simulink model "Mil_Mirror_Subsystem"  (R2018a)
settings: Solver=VariableStepAuto  StartTime=0.0  StopTime=10.0  RelTol=1e-3
undefined symbols (not defined in the file or in its folder): sigbuilder_block
settings Model: Creator=99003191  LastModifiedBy=Anoosha Clarance
settings DataIOCC: ReturnWorkspaceOutputs=on
settings SFSimCC: SimUseLocalCustomCode=on
settings RTWCC: RTWUseLocalCustomCode=on

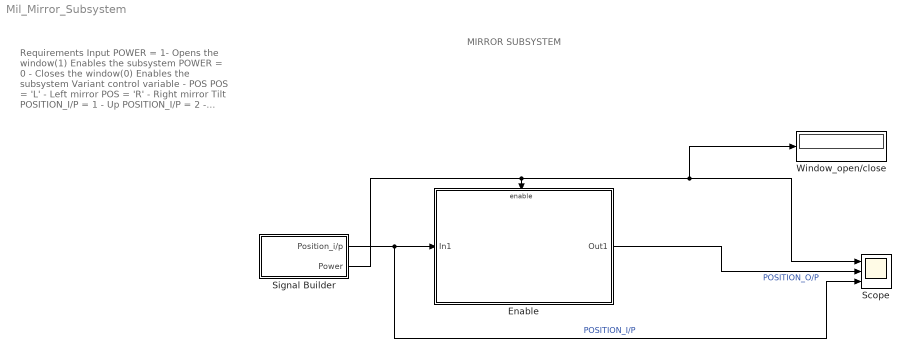
== system Mil_Mirror_Subsystem ==
  note: Requirements
      | Input
      | POWER = 1- Opens the window(1) Enables the subsystem
      | POWER = 0 - Closes the window(0) Enables the subsystem
      | Variant control variable - POS
      | POS = 'L' - Left mirror
      | POS = 'R' - Right mirror
      | Tilt
      | POSITION_I/P = 1 - Up
      | POSITION_I/P = 2 - Down
      | Pan
      | POSITION_I/P = 1 - Right
      | POSITION_I/P = 1 - Left
      |
      | Output
      | Tilt
      | POSITION_O/P = 11 - Left mirror Up
      | POSITION_O/P = 12 - Left mirror Down
      | POSITION_O/P = 21 - Right mirror Up
      | POSITION_O/P = 22 - Right mirror Down
      | Pan
      | POSITION_O/P = 13 - Left mirror Right
      | POSITION_O/P = 14 - Left mirror Left
      | POSITION_O/P = 23 - Right mirror Right
      | POSITION_O/P = 24 - Right mirror Left
  note: MIRROR SUBSYSTEM
  Enable : Subsystem  TreatAsAtomicUnit=on
  Scope : Scope  NumInputPorts=3
  Signal Builder : Subsystem  Tag=STV Subsys  LoadFcn=sigbuilder_block('load');  StartFcn=sigbuilder_block('start');  StopFcn=sigbuilder_block('stop');  ClipboardFcn=sigbuilder_block('clipboard');  mask(Sigbuilder block){tuvar=[0:10]}
      mask help: Simulink:masks:SigbuilderBlock_MD
      mask init:
      | if ~strcmp(get_param(bdroot(gcbh),'SimulationStatus'),'stopped') tuvar = sigbuilder_block('maskInit'); end
      settings: CopyFcn=sigbuilder_block('copy');  DeleteFcn=sigbuilder_block('delete');  ModelCloseFcn=sigbuilder_block('modelClose');  PreSaveFcn=sigbuilder_block('preSave');  PauseFcn=sigbuilder_block('pause');  ContinueFcn=sigbuilder_block('continue');  NameChangeFcn=sigbuilder_block('namechange');  OpenFcn=sigbuilder_block('open',[440.25 156.75 544.5 355.5 ]);  CloseFcn=sigbuilder_block('close');
      mask Display: plot(0, 0, 100, 100,[2, 2, 32, 32, 2], [68, 8, 8, 68, 68],[32, 2], [38, 38], [32, 19, 2],[53, 60, 44], [32, 17, 17, 2],[16, 16, 31, 31]);txt = getActiveGroup(gcbh);text(2, 100, txt,'verticalAlignment', 'top');
  Window_open/close : Display
  wires:
  Signal Builder/1(Position_i/p) -> Scope/3, Enable/1(In1)  "POSITION_I/P"
  Signal Builder/2(Power) -> Window_open/close/1, Scope/1, Enable/Enable
  Enable/1(Out1) -> Scope/2  "POSITION_O/P"

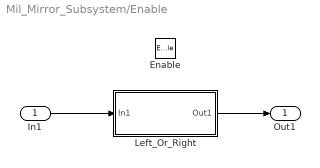
== system Mil_Mirror_Subsystem/Enable ==
  In1 : Inport
  Enable : EnablePort
  Left_Or_Right : Subsystem  Variant=on
  Out1 : Outport
  wires:
  In1/1 -> Left_Or_Right/1(In1)
  Left_Or_Right/1(Out1) -> Out1/1

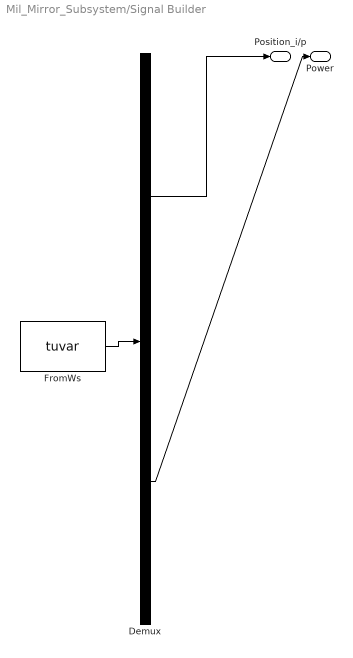
== system Mil_Mirror_Subsystem/Signal Builder ==
  Demux : Demux  Tag=STV Demux  Outputs=2
      settings: DisplayOption=none
  FromWs : FromWorkspace  Tag=STV FromWs  VariableName=tuvar
      SigBuilderData=|
      | common.afterFinalStr = 'Extrapolate'
      | common.sampleTime = 0
      | dataSet.timeRange = [0 10]
      | dataSet.name = 'Group 1'
      | sbobj.Groups.Name = 'Group 1'
      | sbobj.Groups.Signals(1).Name = 'Position_i/p'
      | sbobj.Groups.Signals(1).XData = [0 1 1 2 2 3.02 3.02 4.02 4.02 5 5 5.98 5.98 10]
      | sbobj.Groups.Signals(1).YData = [0 0 3 3 2 2 1 1 3 3 4 4 0 0]
      | sbobj.Groups.Signals(2).Name = 'Power'
      | sbobj.Groups.Signals(2).XData = [0 0.54 0.54 6 6 10]
      | sbobj.Groups.Signals(2).YData = [0 0 1 1 0 0]
  Position_i/p : Outport  Tag=STV Outport
  Power : Outport  Tag=STV Outport  Port=2
  wires:
  Demux/1 -> Position_i/p/1
  FromWs/1 -> Demux/1
  Demux/2 -> Power/1

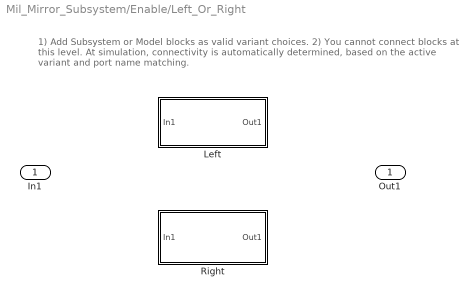
== system Mil_Mirror_Subsystem/Enable/Left_Or_Right ==
  note: 1) Add Subsystem or Model blocks as valid variant choices.
      | 2) You cannot connect blocks at this level. At simulation, connectivity is automatically
      | determined, based on the active variant and port name matching.
  In1 : Inport
  Left : Subsystem  VariantControl=POS == 'L'
  Right : Subsystem  VariantControl=POS == 'R'
  Out1 : Outport

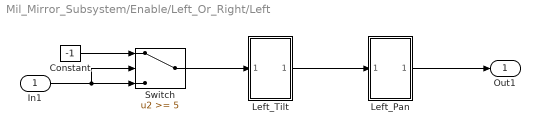
== system Mil_Mirror_Subsystem/Enable/Left_Or_Right/Left ==
  In1 : Inport
  Constant : Constant  Value=-1
  Left_Pan : Subsystem
  Left_Tilt : Subsystem
  Switch : Switch  Threshold=5
  Out1 : Outport
  wires:
  In1/1 -> Switch/2, Switch/3
  Constant/1 -> Switch/1
  Switch/1 -> Left_Tilt/1(In1)
  Left_Tilt/1(Out1) -> Left_Pan/1(In1)
  Left_Pan/1(Out1) -> Out1/1

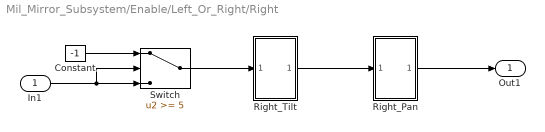
== system Mil_Mirror_Subsystem/Enable/Left_Or_Right/Right ==
  In1 : Inport
  Constant : Constant  Value=-1
  Right_Pan : Subsystem
  Right_Tilt : Subsystem
  Switch : Switch  Threshold=5
  Out1 : Outport
  wires:
  Constant/1 -> Switch/1
  Right_Pan/1(Out1) -> Out1/1
  Switch/1 -> Right_Tilt/1(In1)
  In1/1 -> Switch/2, Switch/3
  Right_Tilt/1(Out1) -> Right_Pan/1(In1)

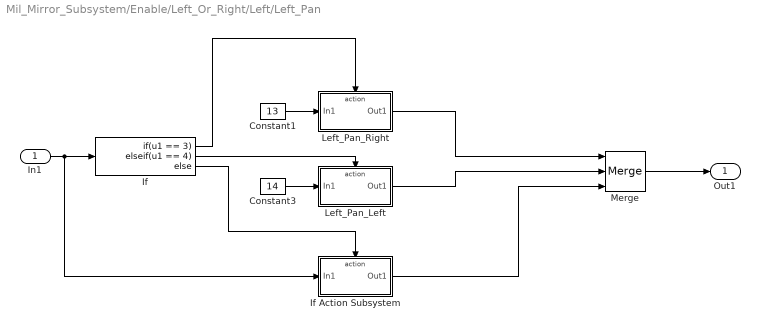
== system Mil_Mirror_Subsystem/Enable/Left_Or_Right/Left/Left_Pan ==
  In1 : Inport
  Constant1 : Constant  Value=13
  Constant3 : Constant  Value=14
  If : If  IfExpression=u1 == 3  ElseIfExpressions=u1 == 4
  If Action Subsystem : Subsystem  TreatAsAtomicUnit=on
  Left_Pan_Left : Subsystem  TreatAsAtomicUnit=on
  Left_Pan_Right : Subsystem  TreatAsAtomicUnit=on
  Merge : Merge  Inputs=3
  Out1 : Outport
  wires:
  Constant1/1 -> Left_Pan_Right/1(In1)
  If/1 -> Left_Pan_Right/Action
  Merge/1 -> Out1/1
  If/2 -> Left_Pan_Left/Action
  Constant3/1 -> Left_Pan_Left/1(In1)
  Left_Pan_Right/1(Out1) -> Merge/1
  Left_Pan_Left/1(Out1) -> Merge/2
  If/3 -> If Action Subsystem/Action
  In1/1 -> If Action Subsystem/1(In1), If/1
  If Action Subsystem/1(Out1) -> Merge/3

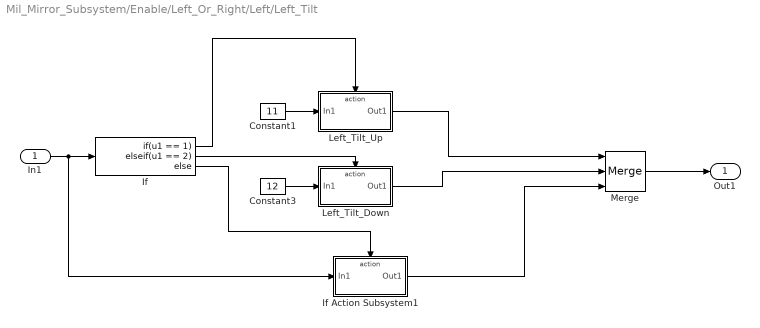
== system Mil_Mirror_Subsystem/Enable/Left_Or_Right/Left/Left_Tilt ==
  In1 : Inport
  Constant1 : Constant  Value=11
  Constant3 : Constant  Value=12
  If : If  IfExpression=u1 == 1  ElseIfExpressions=u1 == 2
  If Action Subsystem1 : Subsystem  TreatAsAtomicUnit=on
  Left_Tilt_Down : Subsystem  TreatAsAtomicUnit=on
  Left_Tilt_Up : Subsystem  TreatAsAtomicUnit=on
  Merge : Merge  Inputs=3
  Out1 : Outport
  wires:
  If/2 -> Left_Tilt_Down/Action
  If/1 -> Left_Tilt_Up/Action
  Constant1/1 -> Left_Tilt_Up/1(In1)
  Left_Tilt_Up/1(Out1) -> Merge/1
  Merge/1 -> Out1/1
  Left_Tilt_Down/1(Out1) -> Merge/2
  Constant3/1 -> Left_Tilt_Down/1(In1)
  If/3 -> If Action Subsystem1/Action
  If Action Subsystem1/1(Out1) -> Merge/3
  In1/1 -> If Action Subsystem1/1(In1), If/1

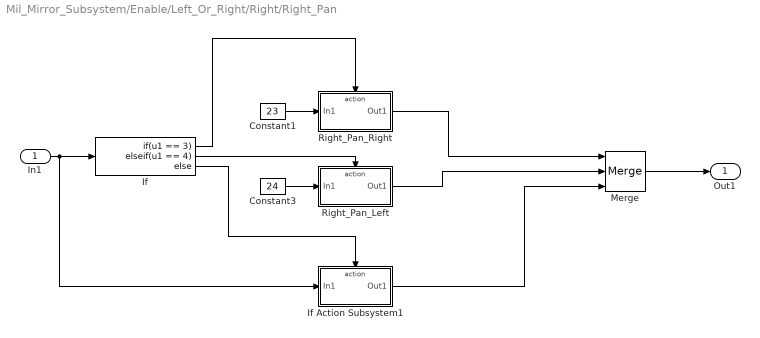
== system Mil_Mirror_Subsystem/Enable/Left_Or_Right/Right/Right_Pan ==
  In1 : Inport
  Constant1 : Constant  Value=23
  Constant3 : Constant  Value=24
  If : If  IfExpression=u1 == 3  ElseIfExpressions=u1 == 4
  If Action Subsystem1 : Subsystem  TreatAsAtomicUnit=on
  Merge : Merge  Inputs=3
  Right_Pan_Left : Subsystem  TreatAsAtomicUnit=on
  Right_Pan_Right : Subsystem  TreatAsAtomicUnit=on
  Out1 : Outport
  wires:
  Constant1/1 -> Right_Pan_Right/1(In1)
  If/1 -> Right_Pan_Right/Action
  Merge/1 -> Out1/1
  If/2 -> Right_Pan_Left/Action
  Constant3/1 -> Right_Pan_Left/1(In1)
  Right_Pan_Right/1(Out1) -> Merge/1
  Right_Pan_Left/1(Out1) -> Merge/2
  In1/1 -> If Action Subsystem1/1(In1), If/1
  If/3 -> If Action Subsystem1/Action
  If Action Subsystem1/1(Out1) -> Merge/3

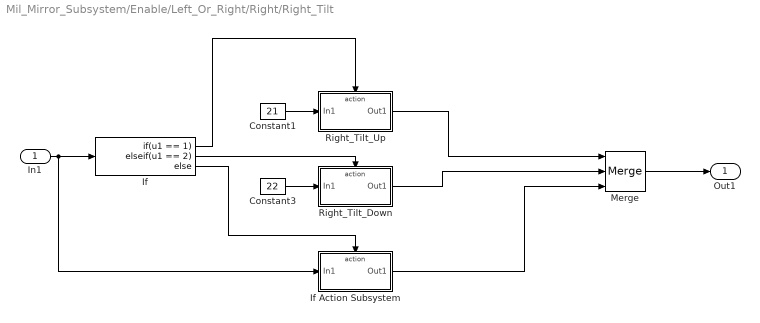
== system Mil_Mirror_Subsystem/Enable/Left_Or_Right/Right/Right_Tilt ==
  In1 : Inport
  Constant1 : Constant  Value=21
  Constant3 : Constant  Value=22
  If : If  IfExpression=u1 == 1  ElseIfExpressions=u1 == 2
  If Action Subsystem : Subsystem  TreatAsAtomicUnit=on
  Merge : Merge  Inputs=3
  Right_Tilt_Down : Subsystem  TreatAsAtomicUnit=on
  Right_Tilt_Up : Subsystem  TreatAsAtomicUnit=on
  Out1 : Outport
  wires:
  If/2 -> Right_Tilt_Down/Action
  If/1 -> Right_Tilt_Up/Action
  Constant1/1 -> Right_Tilt_Up/1(In1)
  Right_Tilt_Up/1(Out1) -> Merge/1
  Merge/1 -> Out1/1
  Right_Tilt_Down/1(Out1) -> Merge/2
  In1/1 -> If Action Subsystem/1(In1), If/1
  Constant3/1 -> Right_Tilt_Down/1(In1)
  If/3 -> If Action Subsystem/Action
  If Action Subsystem/1(Out1) -> Merge/3

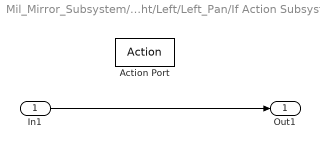
== system Mil_Mirror_Subsystem/Enable/Left_Or_Right/Left/Left_Pan/If Action Subsystem ==
  In1 : Inport
  Action Port : ActionPort
  Out1 : Outport
  wires:
  In1/1 -> Out1/1

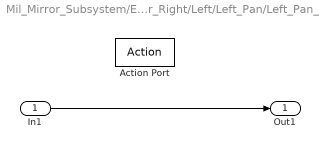
== system Mil_Mirror_Subsystem/Enable/Left_Or_Right/Left/Left_Pan/Left_Pan_Left ==
  In1 : Inport
  Action Port : ActionPort
  Out1 : Outport
  wires:
  In1/1 -> Out1/1

== system Mil_Mirror_Subsystem/Enable/Left_Or_Right/Left/Left_Pan/Left_Pan_Right ==
  In1 : Inport
  Action Port : ActionPort
  Out1 : Outport
  wires:
  In1/1 -> Out1/1

== system Mil_Mirror_Subsystem/Enable/Left_Or_Right/Left/Left_Tilt/If Action Subsystem1 ==
  In1 : Inport
  Action Port : ActionPort
  Out1 : Outport
  wires:
  In1/1 -> Out1/1

== system Mil_Mirror_Subsystem/Enable/Left_Or_Right/Left/Left_Tilt/Left_Tilt_Down ==
  In1 : Inport
  Action Port : ActionPort
  Out1 : Outport
  wires:
  In1/1 -> Out1/1

== system Mil_Mirror_Subsystem/Enable/Left_Or_Right/Left/Left_Tilt/Left_Tilt_Up ==
  In1 : Inport
  Action Port : ActionPort
  Out1 : Outport
  wires:
  In1/1 -> Out1/1

== system Mil_Mirror_Subsystem/Enable/Left_Or_Right/Right/Right_Pan/If Action Subsystem1 ==
  In1 : Inport
  Action Port : ActionPort
  Out1 : Outport
  wires:
  In1/1 -> Out1/1

== system Mil_Mirror_Subsystem/Enable/Left_Or_Right/Right/Right_Pan/Right_Pan_Left ==
  In1 : Inport
  Action Port : ActionPort
  Out1 : Outport
  wires:
  In1/1 -> Out1/1

== system Mil_Mirror_Subsystem/Enable/Left_Or_Right/Right/Right_Pan/Right_Pan_Right ==
  In1 : Inport
  Action Port : ActionPort
  Out1 : Outport
  wires:
  In1/1 -> Out1/1

== system Mil_Mirror_Subsystem/Enable/Left_Or_Right/Right/Right_Tilt/If Action Subsystem ==
  In1 : Inport
  Action Port : ActionPort
  Out1 : Outport
  wires:
  In1/1 -> Out1/1

== system Mil_Mirror_Subsystem/Enable/Left_Or_Right/Right/Right_Tilt/Right_Tilt_Down ==
  In1 : Inport
  Action Port : ActionPort
  Out1 : Outport
  wires:
  In1/1 -> Out1/1

== system Mil_Mirror_Subsystem/Enable/Left_Or_Right/Right/Right_Tilt/Right_Tilt_Up ==
  In1 : Inport
  Action Port : ActionPort
  Out1 : Outport
  wires:
  In1/1 -> Out1/1
